simulink model "CANTXcommunication_1"  (R2024a)
settings: Solver=VariableStepAuto  StartTime=0.0  StopTime=10.0  RelTol=1e-3
undefined symbols (not defined in the file or in its folder): canChannel
libraries: canlib x2, canmsglib x1
settings Model: DataDictionary=BMS_System_dict1.sldd  Creator=hirah  LastModifiedBy=hirah

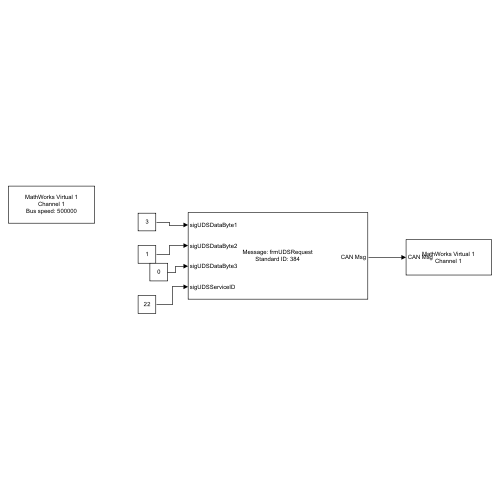
[thumbnail: Simulink's stored preview of the top-level diagram]
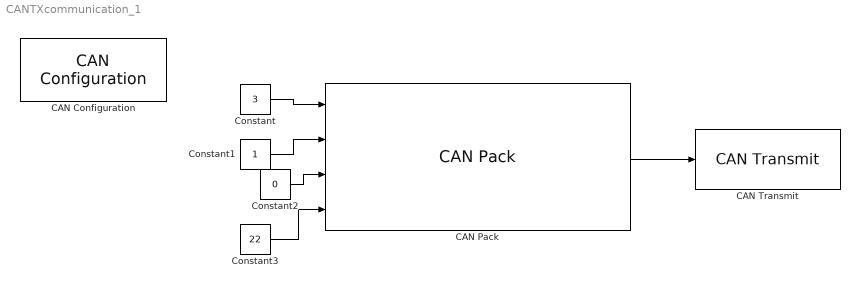
== system CANTXcommunication_1 ==
  CAN Configuration : canlib/CAN Configuration  BlockHandle=708.0002  Device=MathWorks Virtual 1 (Channel 1)  DeviceMenu=MathWorks Virtual 1 (Channel 1)  ObjConstructor=canChannel('MathWorks', 'Virtual 1', 1)  BusSpeed=500000  EnableBitParameters=off  AckMode=Normal
  CAN Pack : canmsglib/CAN Pack  CANdbFile=C:\Users\hirah\Downloads\BMS_CAN_Database (5).dbc  MsgList=frmUDSRequest  MsgName=frmUDSRequest  MsgIDType=Standard (11-bit identifier)  MsgIdentifier=384  MsgLength=8  Remote=off  ApplyMinMax=off  BusOutput=off  SignalInfo={ 'sigUDSDataByte1', '16', '8', 'LE', 'unsigned', 'Standard', '0', '1', '0', '0', '255'; 'sigUDSDataByte2', '24', '8', 'LE', 'unsigned', 'Standard', '0', '1', '0', '0', '255'; 'sigUDSDataByte3', '32', '8', 'LE', 'unsigned', 'Standard', '0', '1', '0', '0', '255'; 'sigUDSServiceID', '0', '8', 'LE', 'unsigned', 'Standard', '0', '1', '0', '0', '255' }
      settings: LibrarySourceBlock=canlib/CAN Pack  DataFormat=manually specified signals
  CAN Transmit : canlib/CAN Transmit  BlockHandle=714.0001  Device=MathWorks Virtual 1 (Channel 1)  DeviceMenu=MathWorks Virtual 1 (Channel 1)  ObjConstructor=canChannel('MathWorks', 'Virtual 1', 1)  EnableEventTransmit=off  EnablePeriodicTransmit=off  MessagePeriod=1.000
  Constant : Constant  Value=3
  Constant1 : Constant
  Constant2 : Constant  Value=0
  Constant3 : Constant  Value=22
  wires:
  CAN Pack/1 -> CAN Transmit/1
  Constant/1 -> CAN Pack/1
  Constant1/1 -> CAN Pack/2
  Constant2/1 -> CAN Pack/3
  Constant3/1 -> CAN Pack/4
